simulink library "IOBlock_Library_TTC580"  (R2021a)
settings: Solver=ode45  StartTime=0.0  StopTime=10.0  RelTol=1e-3
PreLoadFcn:
  | addpath(genpath(fileparts(which('IOBlock_Library_TTC580'))));
  | %addpath(genpath(fileparts(which('IOBlock_Library_TTC580.mdl'))))
  | try
  | addpath(genpath([fileparts(which('IOBlock_Library_TTC580')),'\..\DBC_Importer']));
  | addpath(genpath([fileparts(which('IOBlock_Library_TTC580')),'\..\EEPROM_Importer']));
  | addpath(genpath([fileparts(which('IOBlock_Library_TTC580')),'\..\UserDoc']));
  | catch
  | warning('IOBlock_Library_TTC580: add path to DBC_Importer and EEPROM_Importer manually');
  | end
  | try
  | if exist('..\CustomPackage\scripts\OpenAllPackages.m','file')
  |      run('..\CustomPackage\scripts\OpenAllPackages.m'); %always available, ggf. empty
  | end
  | catch
  | warning('A problem occurred opening automatically the CustomPackage. Please open libraries manually');
  | end
  | try
  | set_param(0,'EditorSmartEditingHotParam','off');
  | catch
  | warning('Simlink preferences for ''Edit key parameter when adding new blocks'' needs to be unchecked manually');
  | end
undefined symbols (not defined in the file or in its folder): ADC_Absolute_10V, ADC_Absolute_32V, ADC_Absolute_5V, ADC_BoardTemp, ADC_ChannelInit, ADC_Current, ADC_Get, ADC_K15_, ADC_Ratiometric_10V, ADC_Ratiometric_5V, ADC_Resistive, ADC_SensorSupply, ADC_UBAT, bit_packing, bit_unpacking, CAN_ConfigMsg, compare2error, compare2FET_PROT_REENABLE, crc32_calc_intern, CRC32_EEPROM_Read, CRC32_EEPROM_Write, DIAG_EnterSafestate, DIAG_Status, DIAG_Status_internal, EEPROM_Mirror, EEPROM_Read, EEPROM_Read_OffsetIn, EEPROM_Read_Raw, EEPROM_Write, EEPROM_Write_OffsetIn, EEPROM_Write_Raw, EnterSafestate, FPU_Handler, Get_DI, Get_DI_VarThreshold, Get_K15_, Get_Pulse_Freq_Curr, Get_Pulse_Freq_Volt, Get_WakeUp, GetDateAndTime, IO_ADC_ResetProtection, IO_Blk_Lib_TTC500, IO_CAN_ReadMsg, IO_CAN_WriteMsg, IO_DI_Get, IO_DI_Init, IO_DI_Init_Var, IO_DO_GetCur, IO_DO_GetVoltage, IO_DO_Init, IO_DO_ResetProtection, IO_DO_Set, IO_Driver_GetSerialNumber, IO_Driver_GetVersionOfDriver, IO_Driver_GetVersionOfFPGA, IO_EEPROM_GetStatus, IO_EEPROM_Init, IO_EEPROM_Read_raw, IO_EEPROM_Write, IO_EEPROM_Write_OffsetIn ... (+73)
libraries: simulink x43
(part 6 of 18)

== system IOBlock_Library_TTC580/UART TTC580 IOlib ==
  UART_Read : Subsystem  LoadFcn=|  mask(UART_Read_Code){SampleTime=-1, ttlib=IO_Blk_Lib_TTC500, ttDescription=UART_Read, tt_iolib_version=0.25, size_of_data=30, Show_additional_information=off, baudrate=115200, dbits=8, par=IO_UART_PARITY_NONE, sbits=1}
      | try
      | %
      | %Upgrade Information - standard BEGIN
      | new_color = 'blue';
      | new_ver = '0.25';
      | act_ver = get_param(gcb,'tt_iolib_version');
      | if not(strcmp(act_ver,new_ver))
      |     disp(['Upgrade block: ',gcb,char(10),'       Version: ',act_ver,' to ',new_ver]);
      |     %switch - case for specific upgrade information e.g. additional parameter required 
      |     %Change appearance and version information
      |     set_param(gcb,'ForegroundColor',new_color);
      |     set_param(gcb,'tt_iolib_version',new_ver);
      | end
      | %Upgrade Information - standard END
      | catch
      | %Standard catch section BEGIN
      | errordlg('An error occurred in a callback of the TTC580-BlockLib. Please open the Diagnostic Viewer for further details');
      | disp(' ');
      | disp('------------------------------------------------------------');
      | disp('An error occurred in a callback of the TTC580-BlockLib.');
      | disp(['Please check the parameters in the mask of ',gcb]);
      | disp('If you do not encounter any violations, then please '); 
      | disp('copy the following lines and report this to support@ttcontrol.com ');
      | disp('<< begin of error message dump >>');
      | disp(['Version of TTC580-BlockLib: ', get_param(gcb,'tt_iolib_version')]);
      | disp(get_param(gcb,'ttDescription'));
      | disp(gcb);
      | x=lasterror;disp(x.message);
      | disp(get_param(gcb,'MaskValues'));
      | disp(version);
      | disp(computer);
      | disp('<< end of error message dump >>');
      | disp('------------------------------------------------------------');
      | disp(' ');
      | %Standard catch section END
      | end
      mask prompts: size_of_data "Size of data array [1 .. 512]"; Show_additional_information "Show additional information"; baudrate "Baud rate [1200 .. 115200]"; dbits "Bits per frame"; par "Parity configuration"; sbits "Stop bits"
      mask help: Read data into uint8 array from serial interface.
      mask init:
      | %
      settings: CopyFcn=%deleted
      mask Help: web([which('usermanual.html'),'#',lower(get_param(gcb,'ttDescription'))])
      mask Callback size_of_data:
      | try
      | sParam = 'size_of_data';
      | vBounds = [1,512];
      | iValue = str2num(get_param(gcb,sParam));
      | if (iValue > vBounds(2))
      |     disp(['Value of ',sParam,' is chosen out of bounds [',num2str(vBounds(1)),'..',num2str(vBounds(2)),'] -> set to maximum possible !!!']);
      |     iValue = vBounds(2); %set to maximum
      |     set_param(gcb,sParam,num2str(iValue));
      | elseif (iValue < vBounds(1))
      |     disp(['Value of ',sParam,' is chosen out of bounds [',num2str(vBounds(1)),'..',num2str(vBounds(2)),'] -> set to minimum possible !!!']);
      |     iValue = vBounds(1); %set to minimum
      |     set_param(gcb,sParam,num2str(iValue));
      | end
      | 
      | catch
      | %Standard catch section BEGIN
      | errordlg('An error occurred in a callback of the TTC580-BlockLib. Please open the Diagnostic Viewer for further details');
      | disp(' ');
      | disp('------------------------------------------------------------');
      | disp('An error occurred in a callback of the TTC580-BlockLib.');
      | disp(['Please check the parameters in the mask of ',gcb]);
      | disp('If you do not encounter any violations, then please ');
      | disp('copy the following lines and report this to support@ttcontrol.com ');
      | disp('<< begin of error message dump >>');
      | disp(['Version of TTC580-BlockLib: ', get_param(gcb,'tt_iolib_version')]);
      | disp(get_param(gcb,'ttDescription'));
      | disp(gcb);
      | x=lasterror;disp(x.message);
      | disp(get_param(gcb,'MaskValues'));
      | disp(version);
      | disp(computer);
      | disp('<< end of error message dump >>');
      | disp('------------------------------------------------------------');
      | disp(' ');
      | %Standard catch section END
      | end
      mask Callback Show_additional_information:
      | try
      | s_ParameterDecision = 'Show_additional_information'; %Deside on this parameter
      | c_ValuesDecision={'off'}; %Positive DescitionValues
      | s_ParameterInvisible = 'baudrate'; %Make this invisible
      | %trim
      | if ischar(s_ParameterInvisible)%if secttion for compatibility reasons of template
      |     cs_ParameterInvisible = {s_ParameterInvisible};
      | else
      |     cs_ParameterInvisible = s_ParameterInvisible;
      | end
      | s_ParameterDecision = strtrim(s_ParameterDecision);
      | c_ValuesDecision = strtrim(c_ValuesDecision);
      | for j=1:length(cs_ParameterInvisible)
      |   s_ParameterInvisible = strtrim(cs_ParameterInvisible{j});
      |   c_MaskVisibilities=get_param(gcb,'MaskVisibilities');
      |   %check consistency
      |   idx=strmatch(s_ParameterInvisible,get_param(gcb,'MaskNames'));
      |   c_MaskVisibilities{idx}='on'; %default
      |     for i = 1: length(c_ValuesDecision)
      |         if ~isempty(strmatch(get_param(gcb, s_ParameterDecision), c_ValuesDecision{i},'exact'))
      |            c_MaskVisibilities{idx}='off';
      |         end
      |     end
      |   set_param(gcb,'MaskVisibilities',c_MaskVisibilities);
      | end
      | s_ParameterDecision = 'Show_additional_information'; %Deside on this parameter
      | c_ValuesDecision={'off'}; %Positive DescitionValues
      | s_ParameterInvisible = 'dbits'; %Make this invisible
      | %trim
      | if ischar(s_ParameterInvisible)%if secttion for compatibility reasons of template
      |     cs_ParameterInvisible = {s_ParameterInvisible};
      | else
      |     cs_ParameterInvisible = s_ParameterInvisible;
      | end
      | s_ParameterDecision = strtrim(s_ParameterDecision);
      | c_ValuesDecision = strtrim(c_ValuesDecision);
      | for j=1:length(cs_ParameterInvisible)
      |   s_ParameterInvisible = strtrim(cs_ParameterInvisible{j});
      |   c_MaskVisibilities=get_param(gcb,'MaskVisibilities');
      |   %check consistency
      |   idx=strmatch(s_ParameterInvisible,get_param(gcb,'MaskNames'));
      |   c_MaskVisibilities{idx}='on'; %default
      |     for i = 1: length(c_ValuesDecision)
      |         if ~isempty(strmatch(get_param(gcb, s_ParameterDecision), c_ValuesDecision{i},'exact'))
      |            c_MaskVisibilities{idx}='off';
      |         end
      |     end
      |   set_param(gcb,'MaskVisibilities',c_MaskVisibilities);
      | end
      | s_ParameterDecision = 'Show_additional_information'; %Deside on this parameter
      | c_ValuesDecision={'off'}; %Positive DescitionValues
      | s_ParameterInvisible = 'par'; %Make this invisible
      | %trim
      | if ischar(s_ParameterInvisible)%if secttion for compatibility reasons of template
      |     cs_ParameterInvisible = {s_ParameterInvisible};
      | else
      |     cs_ParameterInvisible = s_ParameterInvisible;
      | end
      | s_ParameterDecision = strtrim(s_ParameterDecision);
      | c_ValuesDecision = strtrim(c_ValuesDecision);
      | for j=1:length(cs_ParameterInvisible)
      |   s_ParameterInvisible = strtrim(cs_ParameterInvisible{j});
      |   c_MaskVisibilities=get_param(gcb,'MaskVisibilities');
      |   %check consistency
      |   idx=strmatch(s_ParameterInvisible,get_param(gcb,'MaskNames'));
      |   c_MaskVisibilities{idx}='on'; %default
      |     for i = 1: length(c_ValuesDecision)
      |         if ~isempty(strmatch(get_param(gcb, s_ParameterDecision), c_ValuesDecision{i},'exact'))
      |            c_MaskVisibilities{idx}='off';
      |         end
      |     end
      |   set_param(gcb,'MaskVisibilities',c_MaskVisibilities);
      | end
      | s_ParameterDecision = 'Show_additional_information'; %Deside on this parameter
      | c_ValuesDecision={'off'}; %Positive DescitionValues
      | s_ParameterInvisible = 'sbits'; %Make this invisible
      | %trim
      | if ischar(s_ParameterInvisible)%if secttion for compatibility reasons of template
      |     cs_ParameterInvisible = {s_ParameterInvisible};
      | else
      |     cs_ParameterInvisible = s_ParameterInvisible;
      | end
      | s_ParameterDecision = strtrim(s_ParameterDecision);
      | c_ValuesDecision = strtrim(c_ValuesDecision);
      | for j=1:length(cs_ParameterInvisible)
      |   s_ParameterInvisible = strtrim(cs_ParameterInvisible{j});
      |   c_MaskVisibilities=get_param(gcb,'MaskVisibilities');
      |   %check consistency
      |   idx=strmatch(s_ParameterInvisible,get_param(gcb,'MaskNames'));
      |   c_MaskVisibilities{idx}='on'; %default
      |     for i = 1: length(c_ValuesDecision)
      |         if ~isempty(strmatch(get_param(gcb, s_ParameterDecision), c_ValuesDecision{i},'exact'))
      |            c_MaskVisibilities{idx}='off';
      |         end
      |     end
      |   set_param(gcb,'MaskVisibilities',c_MaskVisibilities);
      | end
      | 
      | catch
      | %Standard catch section BEGIN
      | errordlg('An error occurred in a callback of the TTC580-BlockLib. Please open the Diagnostic Viewer for further details');
      | disp(' ');
      | disp('------------------------------------------------------------');
      | disp('An error occurred in a callback of the TTC580-BlockLib.');
      | disp(['Please check the parameters in the mask of ',gcb]);
      | disp('If you do not encounter any violations, then please ');
      | disp('copy the following lines and report this to support@ttcontrol.com ');
      | disp('<< begin of error message dump >>');
      | disp(['Version of TTC580-BlockLib: ', get_param(gcb,'tt_iolib_version')]);
      | disp(get_param(gcb,'ttDescription'));
      | disp(gcb);
      | x=lasterror;disp(x.message);
      | disp(get_param(gcb,'MaskValues'));
      | disp(version);
      | disp(computer);
      | disp('<< end of error message dump >>');
      | disp('------------------------------------------------------------');
      | disp(' ');
      | %Standard catch section END
      | end
      mask Callback baudrate:
      | try
      | sParam = 'baudrate';
      | vBounds = [1200,115200];
      | iValue = str2num(get_param(gcb,sParam));
      | if (iValue > vBounds(2))
      |     disp(['Value of ',sParam,' is chosen out of bounds [',num2str(vBounds(1)),'..',num2str(vBounds(2)),'] -> set to maximum possible !!!']);
      |     iValue = vBounds(2); %set to maximum
      |     set_param(gcb,sParam,num2str(iValue));
      | elseif (iValue < vBounds(1))
      |     disp(['Value of ',sParam,' is chosen out of bounds [',num2str(vBounds(1)),'..',num2str(vBounds(2)),'] -> set to minimum possible !!!']);
      |     iValue = vBounds(1); %set to minimum
      |     set_param(gcb,sParam,num2str(iValue));
      | end
      | 
      | catch
      | %Standard catch section BEGIN
      | errordlg('An error occurred in a callback of the TTC580-BlockLib. Please open the Diagnostic Viewer for further details');
      | disp(' ');
      | disp('------------------------------------------------------------');
      | disp('An error occurred in a callback of the TTC580-BlockLib.');
      | disp(['Please check the parameters in the mask of ',gcb]);
      | disp('If you do not encounter any violations, then please ');
      | disp('copy the following lines and report this to support@ttcontrol.com ');
      | disp('<< begin of error message dump >>');
      | disp(['Version of TTC580-BlockLib: ', get_param(gcb,'tt_iolib_version')]);
      | disp(get_param(gcb,'ttDescription'));
      | disp(gcb);
      | x=lasterror;disp(x.message);
      | disp(get_param(gcb,'MaskValues'));
      | disp(version);
      | disp(computer);
      | disp('<< end of error message dump >>');
      | disp('------------------------------------------------------------');
      | disp(' ');
      | %Standard catch section END
      | end
      mask TypeOptions dbits: 1 | 2 | 3 | 4 | 5 | 6 | 7 | 8
      mask Callback dbits: %
      mask TypeOptions par: IO_UART_PARITY_NONE | IO_UART_PARITY_EVEN | IO_UART_PARITY_ODD
      mask Callback par: %
      mask TypeOptions sbits: 1 | 2
      mask Callback sbits: %
  UART_Write : Subsystem  LoadFcn=|  mask(UART_Write_Code){SampleTime=-1, ttlib=IO_Blk_Lib_TTC500, ttDescription=UART_Write, tt_iolib_version=0.25, Comment=Hello World %d, baudrate=115200, dbits=8, par=IO_UART_PARITY_NONE, sbits=1, max_size=80}
      | try
      | %
      | %Upgrade Information - standard BEGIN
      | new_color = 'blue';
      | new_ver = '0.25';
      | act_ver = get_param(gcb,'tt_iolib_version');
      | if not(strcmp(act_ver,new_ver))
      |     disp(['Upgrade block: ',gcb,char(10),'       Version: ',act_ver,' to ',new_ver]);
      |     %switch - case for specific upgrade information e.g. additional parameter required 
      |     %Change appearance and version information
      |     set_param(gcb,'ForegroundColor',new_color);
      |     set_param(gcb,'tt_iolib_version',new_ver);
      | end
      | %Upgrade Information - standard END
      | catch
      | %Standard catch section BEGIN
      | errordlg('An error occurred in a callback of the TTC580-BlockLib. Please open the Diagnostic Viewer for further details');
      | disp(' ');
      | disp('------------------------------------------------------------');
      | disp('An error occurred in a callback of the TTC580-BlockLib.');
      | disp(['Please check the parameters in the mask of ',gcb]);
      | disp('If you do not encounter any violations, then please '); 
      | disp('copy the following lines and report this to support@ttcontrol.com ');
      | disp('<< begin of error message dump >>');
      | disp(['Version of TTC580-BlockLib: ', get_param(gcb,'tt_iolib_version')]);
      | disp(get_param(gcb,'ttDescription'));
      | disp(gcb);
      | x=lasterror;disp(x.message);
      | disp(get_param(gcb,'MaskValues'));
      | disp(version);
      | disp(computer);
      | disp('<< end of error message dump >>');
      | disp('------------------------------------------------------------');
      | disp(' ');
      | %Standard catch section END
      | end
      mask prompts: baudrate "Baud rate (1200..115200)"; dbits "Bits per frame"; par "Parity configuration"; sbits "Stop bits"
      mask help: Writes multiple value with comment to UART interface
      mask init:
      | try
      | %%%calculate derate
      | if evalin('base','~exist(''DERATE_PRINTF'')') || evalin('base','~isnumeric(DERATE_PRINTF)')
      |    derate_val = 100;
      | else
      |    derate_val = evalin('base','real(ceil(DERATE_PRINTF))');
      | end
      | catch
      | %Standard catch section BEGIN
      | errordlg('An error occurred in a callback of the TTC580-BlockLib. Please open the Diagnostic Viewer for further details');
      | disp(' ');
      | disp('------------------------------------------------------------');
      | disp('An error occurred in a callback of the TTC580-BlockLib.');
      | disp(['Please check the parameters in the mask of ',gcb]);
      | disp('If you do not encounter any violations, then please '); 
      | disp('copy the following lines and report this to support@ttcontrol.com ');
      | disp('<< begin of error message dump >>');
      | disp(['Version of TTC580-BlockLib: ', get_param(gcb,'tt_iolib_version')]);
      | disp(get_param(gcb,'ttDescription'));
      | disp(gcb);
      | x=lasterror;disp(x.message);
      | disp(get_param(gcb,'MaskValues'));
      | disp(version);
      | disp(computer);
      | disp('<< end of error message dump >>');
      | disp('------------------------------------------------------------');
      | disp(' ');
      | %Standard catch section END
      | end
      settings: CopyFcn=%deleted
      mask Help: web([which('usermanual.html'),'#',lower(get_param(gcb,'ttDescription'))])
      mask Callback Comment:
      | try
      | sComment = get_param(gcb,'Comment');
      | if any(uint8(sComment)==10) %CR detected
      |     warning(['The parameter Comment: ',sComment,' contains a CR-Character try to repair ....']);
      |     sComment_new = strrep(sComment,char(10),' '); %remove CR
      |     set_param(gcb,'Comment',sComment_new);
      |     disp('Repair for the parameter Comment successfully completed, please save your model.');
      | end
      | catch
      | %Standard catch section BEGIN
      | errordlg('An error occurred in a callback of the TTC580-BlockLib. Please open the Diagnostic Viewer for further details');
      | disp(' ');
      | disp('------------------------------------------------------------');
      | disp('An error occurred in a callback of the TTC580-BlockLib.');
      | disp(['Please check the parameters in the mask of ',gcb]);
      | disp('If you do not encounter any violations, then please ');
      | disp('copy the following lines and report this to support@ttcontrol.com ');
      | disp('<< begin of error message dump >>');
      | disp(['Version of TTC580-BlockLib: ', get_param(gcb,'tt_iolib_version')]);
      | disp(get_param(gcb,'ttDescription'));
      | disp(gcb);
      | x=lasterror;disp(x.message);
      | disp(get_param(gcb,'MaskValues'));
      | disp(version);
      | disp(computer);
      | disp('<< end of error message dump >>');
      | disp('------------------------------------------------------------');
      | disp(' ');
      | %Standard catch section END
      | end
      mask Callback baudrate:
      | try
      | sParam = 'baudrate';
      | vBounds = [1200,115200];
      | iValue = str2num(get_param(gcb,sParam));
      | if (iValue > vBounds(2))
      |     disp(['Value of ',sParam,' is chosen out of bounds [',num2str(vBounds(1)),'..',num2str(vBounds(2)),'] -> set to maximum possible !!!']);
      |     iValue = vBounds(2); %set to maximum
      |     set_param(gcb,sParam,num2str(iValue));
      | elseif (iValue < vBounds(1))
      |     disp(['Value of ',sParam,' is chosen out of bounds [',num2str(vBounds(1)),'..',num2str(vBounds(2)),'] -> set to minimum possible !!!']);
      |     iValue = vBounds(1); %set to minimum
      |     set_param(gcb,sParam,num2str(iValue));
      | end
      | 
      | catch
      | %Standard catch section BEGIN
      | errordlg('An error occurred in a callback of the TTC580-BlockLib. Please open the Diagnostic Viewer for further details');
      | disp(' ');
      | disp('------------------------------------------------------------');
      | disp('An error occurred in a callback of the TTC580-BlockLib.');
      | disp(['Please check the parameters in the mask of ',gcb]);
      | disp('If you do not encounter any violations, then please ');
      | disp('copy the following lines and report this to support@ttcontrol.com ');
      | disp('<< begin of error message dump >>');
      | disp(['Version of TTC580-BlockLib: ', get_param(gcb,'tt_iolib_version')]);
      | disp(get_param(gcb,'ttDescription'));
      | disp(gcb);
      | x=lasterror;disp(x.message);
      | disp(get_param(gcb,'MaskValues'));
      | disp(version);
      | disp(computer);
      | disp('<< end of error message dump >>');
      | disp('------------------------------------------------------------');
      | disp(' ');
      | %Standard catch section END
      | end
      mask TypeOptions dbits: 1 | 2 | 3 | 4 | 5 | 6 | 7 | 8
      mask Callback dbits: %
      mask TypeOptions par: IO_UART_PARITY_NONE | IO_UART_PARITY_EVEN | IO_UART_PARITY_ODD
      mask Callback par: %
      mask TypeOptions sbits: 1 | 2
      mask Callback sbits: %
      mask Callback max_size: %
  Write_RS232_ : Subsystem  LoadFcn=|  TreatAsAtomicUnit=on  mask(Write_RS232__Code){SampleTime=-1, ttlib=IO_Blk_Lib_TTC500, ttDescription=Write_RS232_, tt_iolib_version=0.25, Comment=Hello World =}
      | try
      | %specific upgrade to 0.14
      | if (0.14 > str2num(get_param(gcb,'tt_iolib_version'))) || (0.8 == str2num(get_param(gcb,'tt_iolib_version')))
      |     warning('off','Simulink:SL_RefBlockUnknownParameter');   %R2007b: no parameter.mode available in mask any more
      |     warning('off','Simulink:blocks:RefBlockUnknownParameter'); %same for R2014
      | end
      | %Upgrade Information - standard BEGIN
      | new_color = 'blue';
      | new_ver = '0.25';
      | act_ver = get_param(gcb,'tt_iolib_version');
      | if not(strcmp(act_ver,new_ver))
      |     disp(['Upgrade block: ',gcb,char(10),'       Version: ',act_ver,' to ',new_ver]);
      |     %switch - case for specific upgrade information e.g. additional parameter required 
      |     %Change appearance and version information
      |     set_param(gcb,'ForegroundColor',new_color);
      |     set_param(gcb,'tt_iolib_version',new_ver);
      | end
      | %Upgrade Information - standard END
      | catch
      | %Standard catch section BEGIN
      | errordlg('An error occurred in a callback of the TTC580-BlockLib. Please open the Diagnostic Viewer for further details');
      | disp(' ');
      | disp('------------------------------------------------------------');
      | disp('An error occurred in a callback of the TTC580-BlockLib.');
      | disp(['Please check the parameters in the mask of ',gcb]);
      | disp('If you do not encounter any violations, then please '); 
      | disp('copy the following lines and report this to support@ttcontrol.com ');
      | disp('<< begin of error message dump >>');
      | disp(['Version of TTC580-BlockLib: ', get_param(gcb,'tt_iolib_version')]);
      | disp(get_param(gcb,'ttDescription'));
      | disp(gcb);
      | x=lasterror;disp(x.message);
      | disp(get_param(gcb,'MaskValues'));
      | disp(version);
      | disp(computer);
      | disp('<< end of error message dump >>');
      | disp('------------------------------------------------------------');
      | disp(' ');
      | %Standard catch section END
      | end
      mask help: Writes a value with comment to UART interface
      mask init:
      | try
      | sComment_trim = strtrim(get_param(gcb,'Comment'));
      | if ~isempty(strfind(sComment_trim,'%'))
      |     error(['In ',gcb,' there is a "%" that indicates the usage of format specifiers -> please delete this "%" ']);
      | elseif ~isempty(strfind(sComment_trim,'\'))
      |     error(['In ',gcb,' there is a "\" (backslash) that indicates the usage of an escape sequence -> please delete this "\" ']);
      | elseif ~isempty(strfind(sComment_trim,'"'))
      |     error(['In ',gcb,' the comment string shall not have any quotes -> please delete all quotes ']);
      | end
      | %%%calculate derate
      | if evalin('base','~exist(''DERATE_PRINTF'')') || evalin('base','~isnumeric(DERATE_PRINTF)')
      |    derate_val = 100;
      | else
      |    derate_val = evalin('base','real(ceil(DERATE_PRINTF))');
      | end
      | catch
      | %Standard catch section BEGIN
      | errordlg('An error occurred in a callback of the TTC580-BlockLib. Please open the Diagnostic Viewer for further details');
      | disp(' ');
      | disp('------------------------------------------------------------');
      | disp('An error occurred in a callback of the TTC580-BlockLib.');
      | disp(['Please check the parameters in the mask of ',gcb]);
      | disp('If you do not encounter any violations, then please '); 
      | disp('copy the following lines and report this to support@ttcontrol.com ');
      | disp('<< begin of error message dump >>');
      | disp(['Version of TTC580-BlockLib: ', get_param(gcb,'tt_iolib_version')]);
      | disp(get_param(gcb,'ttDescription'));
      | disp(gcb);
      | x=lasterror;disp(x.message);
      | disp(get_param(gcb,'MaskValues'));
      | disp(version);
      | disp(computer);
      | disp('<< end of error message dump >>');
      | disp('------------------------------------------------------------');
      | disp(' ');
      | %Standard catch section END
      | end
      settings: CopyFcn=%deleted  RTWSystemCode=Inline
      mask Help: web([which('usermanual.html'),'#',lower(get_param(gcb,'ttDescription'))])
      mask Callback Comment:
      | try
      | sComment = get_param(gcb,'Comment');
      | if any(uint8(sComment)==10) %CR detected
      |     warning(['The parameter Comment: ',sComment,' contains a CR-Character try to repair ....']);
      |     sComment_new = strrep(sComment,char(10),''); %remove CR
      |     set_param(gcb,'Comment',sComment_new);
      |     disp('Repair for the parameter Comment successfully completed, please save your model.');
      | end
      | catch
      | %Standard catch section BEGIN
      | errordlg('An error occurred in a callback of the TTC580-BlockLib. Please open the Diagnostic Viewer for further details');
      | disp(' ');
      | disp('------------------------------------------------------------');
      | disp('An error occurred in a callback of the TTC580-BlockLib.');
      | disp(['Please check the parameters in the mask of ',gcb]);
      | disp('If you do not encounter any violations, then please ');
      | disp('copy the following lines and report this to support@ttcontrol.com ');
      | disp('<< begin of error message dump >>');
      | disp(['Version of TTC580-BlockLib: ', get_param(gcb,'tt_iolib_version')]);
      | disp(get_param(gcb,'ttDescription'));
      | disp(gcb);
      | x=lasterror;disp(x.message);
      | disp(get_param(gcb,'MaskValues'));
      | disp(version);
      | disp(computer);
      | disp('<< end of error message dump >>');
      | disp('------------------------------------------------------------');
      | disp(' ');
      | %Standard catch section END
      | end
  Write_RS232_green : Subsystem  Priority=620  LoadFcn=|  TreatAsAtomicUnit=on  mask(Write_RS232_Green_Code){SampleTime=-1, ttlib=IO_Blk_Lib_TTC500, ttDescription=Write_RS232_green, tt_iolib_version=0.25, Comment=Hello World (green) =}
      | try
      | %specific upgrade to 0.14
      | if (0.14 > str2num(get_param(gcb,'tt_iolib_version'))) || (0.8 == str2num(get_param(gcb,'tt_iolib_version')))
      |     warning('off','Simulink:SL_RefBlockUnknownParameter');   %R2007b: no parameter.mode available in mask any more
      |     warning('off','Simulink:blocks:RefBlockUnknownParameter'); %same for R2014
      | end
      | %Upgrade Information - standard BEGIN
      | new_color = 'blue';
      | new_ver = '0.25';
      | act_ver = get_param(gcb,'tt_iolib_version');
      | if not(strcmp(act_ver,new_ver))
      |     disp(['Upgrade block: ',gcb,char(10),'       Version: ',act_ver,' to ',new_ver]);
      |     %switch - case for specific upgrade information e.g. additional parameter required 
      |     %Change appearance and version information
      |     set_param(gcb,'ForegroundColor',new_color);
      |     set_param(gcb,'tt_iolib_version',new_ver);
      | end
      | %Upgrade Information - standard END
      | catch
      | %Standard catch section BEGIN
      | errordlg('An error occurred in a callback of the TTC580-BlockLib. Please open the Diagnostic Viewer for further details');
      | disp(' ');
      | disp('------------------------------------------------------------');
      | disp('An error occurred in a callback of the TTC580-BlockLib.');
      | disp(['Please check the parameters in the mask of ',gcb]);
      | disp('If you do not encounter any violations, then please '); 
      | disp('copy the following lines and report this to support@ttcontrol.com ');
      | disp('<< begin of error message dump >>');
      | disp(['Version of TTC580-BlockLib: ', get_param(gcb,'tt_iolib_version')]);
      | disp(get_param(gcb,'ttDescription'));
      | disp(gcb);
      | x=lasterror;disp(x.message);
      | disp(get_param(gcb,'MaskValues'));
      | disp(version);
      | disp(computer);
      | disp('<< end of error message dump >>');
      | disp('------------------------------------------------------------');
      | disp(' ');
      | %Standard catch section END
      | end
      mask help: Triggered writing of a non zero value with green comment to UART interface
      mask init: same as IOBlock_Library_TTC580/UART TTC580 IOlib/Write_RS232_
      settings: CopyFcn=%deleted  RTWSystemCode=Inline
      mask Help: web([which('usermanual.html'),'#',lower(get_param(gcb,'ttDescription'))])
      mask Callback Comment:
      | try
      | sComment = get_param(gcb,'Comment');
      | if any(uint8(sComment)==10) %CR detected
      |     warning(['The parameter Comment: ',sComment,' contains a CR-Character try to repair ....']);
      |     sComment_new = strrep(sComment,char(10),''); %remove CR
      |     set_param(gcb,'Comment',sComment_new);
      |     disp('Repair for the parameter Comment successfully completed, please save your model.');
      | end
      | catch
      | %Standard catch section BEGIN
      | errordlg('An error occurred in a callback of the TTC580-BlockLib. Please open the Diagnostic Viewer for further details');
      | disp(' ');
      | disp('------------------------------------------------------------');
      | disp('An error occurred in a callback of the TTC580-BlockLib.');
      | disp(['Please check the parameters in the mask of ',gcb]);
      | disp('If you do not encounter any violations, then please ');
      | disp('copy the following lines and report this to support@ttcontrol.com ');
      | disp('<< begin of error message dump >>');
      | disp(['Version of TTC580-BlockLib: ', get_param(gcb,'tt_iolib_version')]);
      | disp(get_param(gcb,'ttDescription'));
      | disp(gcb);
      | x=lasterror;disp(x.message);
      | disp(get_param(gcb,'MaskValues'));
      | disp(version);
      | disp(computer);
      | disp('<< end of error message dump >>');
      | disp('------------------------------------------------------------');
      | disp(' ');
      | %Standard catch section END
      | end
  Write_RS232_red : Subsystem  Priority=620  LoadFcn=|  TreatAsAtomicUnit=on  mask(Write_RS232_Red_Code){SampleTime=-1, ttlib=IO_Blk_Lib_TTC500, ttDescription=Write_RS232_red, tt_iolib_version=0.25, Comment=Hello World (red) =}
      | try
      | %specific upgrade to 0.14
      | if (0.14 > str2num(get_param(gcb,'tt_iolib_version'))) || (0.8 == str2num(get_param(gcb,'tt_iolib_version')))
      |     warning('off','Simulink:SL_RefBlockUnknownParameter');   %R2007b: no parameter.mode available in mask any more
      |     warning('off','Simulink:blocks:RefBlockUnknownParameter'); %same for R2014
      | end
      | %Upgrade Information - standard BEGIN
      | new_color = 'blue';
      | new_ver = '0.25';
      | act_ver = get_param(gcb,'tt_iolib_version');
      | if not(strcmp(act_ver,new_ver))
      |     disp(['Upgrade block: ',gcb,char(10),'       Version: ',act_ver,' to ',new_ver]);
      |     %switch - case for specific upgrade information e.g. additional parameter required 
      |     %Change appearance and version information
      |     set_param(gcb,'ForegroundColor',new_color);
      |     set_param(gcb,'tt_iolib_version',new_ver);
      | end
      | %Upgrade Information - standard END
      | catch
      | %Standard catch section BEGIN
      | errordlg('An error occurred in a callback of the TTC580-BlockLib. Please open the Diagnostic Viewer for further details');
      | disp(' ');
      | disp('------------------------------------------------------------');
      | disp('An error occurred in a callback of the TTC580-BlockLib.');
      | disp(['Please check the parameters in the mask of ',gcb]);
      | disp('If you do not encounter any violations, then please '); 
      | disp('copy the following lines and report this to support@ttcontrol.com ');
      | disp('<< begin of error message dump >>');
      | disp(['Version of TTC580-BlockLib: ', get_param(gcb,'tt_iolib_version')]);
      | disp(get_param(gcb,'ttDescription'));
      | disp(gcb);
      | x=lasterror;disp(x.message);
      | disp(get_param(gcb,'MaskValues'));
      | disp(version);
      | disp(computer);
      | disp('<< end of error message dump >>');
      | disp('------------------------------------------------------------');
      | disp(' ');
      | %Standard catch section END
      | end
      mask help: Triggered writing of a non zero value with red comment to UART interface
      mask init: same as IOBlock_Library_TTC580/UART TTC580 IOlib/Write_RS232_
      settings: CopyFcn=%deleted  RTWSystemCode=Inline
      mask Help: web([which('usermanual.html'),'#',lower(get_param(gcb,'ttDescription'))])
      mask Callback Comment:
      | try
      | sComment = get_param(gcb,'Comment');
      | if any(uint8(sComment)==10) %CR detected
      |     warning(['The parameter Comment: ',sComment,' contains a CR-Character try to repair ....']);
      |     sComment_new = strrep(sComment,char(10),''); %remove CR
      |     set_param(gcb,'Comment',sComment_new);
      |     disp('Repair for the parameter Comment successfully completed, please save your model.');
      | end
      | catch
      | %Standard catch section BEGIN
      | errordlg('An error occurred in a callback of the TTC580-BlockLib. Please open the Diagnostic Viewer for further details');
      | disp(' ');
      | disp('------------------------------------------------------------');
      | disp('An error occurred in a callback of the TTC580-BlockLib.');
      | disp(['Please check the parameters in the mask of ',gcb]);
      | disp('If you do not encounter any violations, then please ');
      | disp('copy the following lines and report this to support@ttcontrol.com ');
      | disp('<< begin of error message dump >>');
      | disp(['Version of TTC580-BlockLib: ', get_param(gcb,'tt_iolib_version')]);
      | disp(get_param(gcb,'ttDescription'));
      | disp(gcb);
      | x=lasterror;disp(x.message);
      | disp(get_param(gcb,'MaskValues'));
      | disp(version);
      | disp(computer);
      | disp('<< end of error message dump >>');
      | disp('------------------------------------------------------------');
      | disp(' ');
      | %Standard catch section END
      | end

== system IOBlock_Library_TTC580/ADC Blocks TTC580 IOlib/ADC_Absolute_10V ==
  ADC_ChannelInit : Subsystem  LoadFcn=|  mask(ADC_ChannelInit_Code){SampleTime=-1, ttlib=IO_Blk_Lib_TTC500, ttDescription=ADC_ChannelInit, tt_iolib_version=0.19, adc_channel=adc_channel, adc_type=adc_type, range=range, pupd=pupd, sensor_supply=sensor_supply, safety_conf=NULL}
      | try
      | %
      | %Upgrade Information - standard BEGIN
      | new_color = 'blue';
      | new_ver = '0.19';
      | act_ver = get_param(gcb,'tt_iolib_version');
      | if not(strcmp(act_ver,new_ver))
      |     disp(['Upgrade block: ',gcb,char(10),'       Version: ',act_ver,' -> ',new_ver]);
      |     %switch - case for specific upgrade information e.g. additional parameter required 
      |     %Change appearance and version information
      |     set_param(gcb,'ForegroundColor',new_color);
      |     set_param(gcb,'tt_iolib_version',new_ver);
      | end
      | %Upgrade Information - standard END
      | catch
      | %Standard catch section BEGIN 
      | disp(' ');
      | disp('------------------------------------------------------------');
      | disp('An error occurred in a callback of the TTC580-BlockLib.');
      | disp(['Please check the parameters in the mask of ',gcb]);
      | disp('If you do not encounter any violations, then please '); 
      | disp('copy the following lines and report this to support@ttcontrol.com ');
      | disp('<< begin of error message dump >>');
      | disp(['Version of TTC580-BlockLib: ', get_param(gcb,'tt_iolib_version')]);
      | disp(get_param(gcb,'ttDescription'));
      | disp(gcb);
      | x=lasterror;disp(x.message);
      | disp(get_param(gcb,'MaskValues'));
      | disp(version);
      | disp(computer);
      | disp('<< end of error message dump >>');
      | disp('------------------------------------------------------------');
      | disp(' ');
      | %Standard catch section END
      | end
      mask help: Setup one ADC channel.
      mask init:
      | %
      settings: CopyFcn=%deleted
      mask Help: web(which('IO_ADC.h'))
      mask Callback adc_channel: %
      mask Callback adc_type: %
      mask Callback range: %
      mask Callback pupd: %
      mask Callback sensor_supply: %
      mask Callback safety_conf: %
  ADC_Get : Subsystem  LoadFcn=|  mask(ADC_Get_Code){SampleTime=-1, ttlib=IO_Blk_Lib_TTC500, ttDescription=ADC_Get, tt_iolib_version=0.19, adc_channel=adc_channel}
      | try
      | %
      | %Upgrade Information - standard BEGIN
      | new_color = 'blue';
      | new_ver = '0.19';
      | act_ver = get_param(gcb,'tt_iolib_version');
      | if not(strcmp(act_ver,new_ver))
      |     disp(['Upgrade block: ',gcb,char(10),'       Version: ',act_ver,' -> ',new_ver]);
      |     %switch - case for specific upgrade information e.g. additional parameter required 
      |     %Change appearance and version information
      |     set_param(gcb,'ForegroundColor',new_color);
      |     set_param(gcb,'tt_iolib_version',new_ver);
      | end
      | %Upgrade Information - standard END
      | catch
      | %Standard catch section BEGIN 
      | disp(' ');
      | disp('------------------------------------------------------------');
      | disp('An error occurred in a callback of the TTC580-BlockLib.');
      | disp(['Please check the parameters in the mask of ',gcb]);
      | disp('If you do not encounter any violations, then please '); 
      | disp('copy the following lines and report this to support@ttcontrol.com ');
      | disp('<< begin of error message dump >>');
      | disp(['Version of TTC580-BlockLib: ', get_param(gcb,'tt_iolib_version')]);
      | disp(get_param(gcb,'ttDescription'));
      | disp(gcb);
      | x=lasterror;disp(x.message);
      | disp(get_param(gcb,'MaskValues'));
      | disp(version);
      | disp(computer);
      | disp('<< end of error message dump >>');
      | disp('------------------------------------------------------------');
      | disp(' ');
      | %Standard catch section END
      | end
      mask help: Returns the value of the given ADC channel.
      mask init:
      | %
      settings: CopyFcn=%deleted
      mask Help: web(which('IO_ADC.h'))
      mask Callback adc_channel: %
  PWM_Init : Terminator
  PWM_Init1 : Terminator
  ErrorCode : Outport  VectorParamsAs1DForOutWhenUnconnected=off
  adc_value : Outport  Port=2  VectorParamsAs1DForOutWhenUnconnected=off
  wires:
  ADC_ChannelInit/1(ErrorCode) -> PWM_Init/1
  ADC_Get/3(fresh) -> PWM_Init1/1
  ADC_Get/1(ErrorCode) -> ErrorCode/1
  ADC_Get/2(adc_value) -> adc_value/1

== system IOBlock_Library_TTC580/ADC Blocks TTC580 IOlib/ADC_Absolute_32V ==
  ADC_ChannelInit : Subsystem  LoadFcn=|  mask(ADC_ChannelInit_Code){SampleTime=-1, ttlib=IO_Blk_Lib_TTC500, ttDescription=ADC_ChannelInit, tt_iolib_version=0.19, adc_channel=adc_channel, adc_type=adc_type, range=range, pupd=pupd, sensor_supply=sensor_supply, safety_conf=NULL}
      | try
      | %
      | %Upgrade Information - standard BEGIN
      | new_color = 'blue';
      | new_ver = '0.19';
      | act_ver = get_param(gcb,'tt_iolib_version');
      | if not(strcmp(act_ver,new_ver))
      |     disp(['Upgrade block: ',gcb,char(10),'       Version: ',act_ver,' -> ',new_ver]);
      |     %switch - case for specific upgrade information e.g. additional parameter required 
      |     %Change appearance and version information
      |     set_param(gcb,'ForegroundColor',new_color);
      |     set_param(gcb,'tt_iolib_version',new_ver);
      | end
      | %Upgrade Information - standard END
      | catch
      | %Standard catch section BEGIN 
      | disp(' ');
      | disp('------------------------------------------------------------');
      | disp('An error occurred in a callback of the TTC580-BlockLib.');
      | disp(['Please check the parameters in the mask of ',gcb]);
      | disp('If you do not encounter any violations, then please '); 
      | disp('copy the following lines and report this to support@ttcontrol.com ');
      | disp('<< begin of error message dump >>');
      | disp(['Version of TTC580-BlockLib: ', get_param(gcb,'tt_iolib_version')]);
      | disp(get_param(gcb,'ttDescription'));
      | disp(gcb);
      | x=lasterror;disp(x.message);
      | disp(get_param(gcb,'MaskValues'));
      | disp(version);
      | disp(computer);
      | disp('<< end of error message dump >>');
      | disp('------------------------------------------------------------');
      | disp(' ');
      | %Standard catch section END
      | end
      mask help: Setup one ADC channel.
      mask init:
      | %
      settings: CopyFcn=%deleted
      mask Help: web(which('IO_ADC.h'))
      mask Callback adc_channel: %
      mask Callback adc_type: %
      mask Callback range: %
      mask Callback pupd: %
      mask Callback sensor_supply: %
      mask Callback safety_conf: %
  ADC_Get : Subsystem  LoadFcn=|  mask(ADC_Get_Code){SampleTime=-1, ttlib=IO_Blk_Lib_TTC500, ttDescription=ADC_Get, tt_iolib_version=0.19, adc_channel=adc_channel}
      | try
      | %
      | %Upgrade Information - standard BEGIN
      | new_color = 'blue';
      | new_ver = '0.19';
      | act_ver = get_param(gcb,'tt_iolib_version');
      | if not(strcmp(act_ver,new_ver))
      |     disp(['Upgrade block: ',gcb,char(10),'       Version: ',act_ver,' -> ',new_ver]);
      |     %switch - case for specific upgrade information e.g. additional parameter required 
      |     %Change appearance and version information
      |     set_param(gcb,'ForegroundColor',new_color);
      |     set_param(gcb,'tt_iolib_version',new_ver);
      | end
      | %Upgrade Information - standard END
      | catch
      | %Standard catch section BEGIN 
      | disp(' ');
      | disp('------------------------------------------------------------');
      | disp('An error occurred in a callback of the TTC580-BlockLib.');
      | disp(['Please check the parameters in the mask of ',gcb]);
      | disp('If you do not encounter any violations, then please '); 
      | disp('copy the following lines and report this to support@ttcontrol.com ');
      | disp('<< begin of error message dump >>');
      | disp(['Version of TTC580-BlockLib: ', get_param(gcb,'tt_iolib_version')]);
      | disp(get_param(gcb,'ttDescription'));
      | disp(gcb);
      | x=lasterror;disp(x.message);
      | disp(get_param(gcb,'MaskValues'));
      | disp(version);
      | disp(computer);
      | disp('<< end of error message dump >>');
      | disp('------------------------------------------------------------');
      | disp(' ');
      | %Standard catch section END
      | end
      mask help: Returns the value of the given ADC channel.
      mask init:
      | %
      settings: CopyFcn=%deleted
      mask Help: web(which('IO_ADC.h'))
      mask Callback adc_channel: %
  PWM_Init : Terminator
  PWM_Init1 : Terminator
  ErrorCode : Outport  VectorParamsAs1DForOutWhenUnconnected=off
  adc_value : Outport  Port=2  VectorParamsAs1DForOutWhenUnconnected=off
  wires:
  ADC_ChannelInit/1(ErrorCode) -> PWM_Init/1
  ADC_Get/3(fresh) -> PWM_Init1/1
  ADC_Get/1(ErrorCode) -> ErrorCode/1
  ADC_Get/2(adc_value) -> adc_value/1
